simulink model "battery_system_CV_PID"  (R2022a)
settings: Solver=VariableStepAuto  StartTime=0.0  StopTime=10.0  RelTol=1e-3
model workspace (MAT data in the model file):
  AN : object (value not decoded)
  C = [0 0 -0.999999993923 0 0 0 0 0 0 0 0 0 ... (355 elements, 1x355)]
  CA : object (value not decoded)
  CONS : object (value not decoded)
  CV_ref = 3.74905480499
  EL : object (value not decoded)
  FLAG : object (value not decoded)
  K_D = 0
  K_I = -7437.93380511
  K_P = 0
  K_algb = [0 0 0 0 0 0 0 0 0 0 0 0 ... (126025 elements, 355x355)]
  M_cross = [1 0 0 0 0 0 0 0 0 0 0 0 ... (126025 elements, 355x355)]
  N : object (value not decoded)
  P : object (value not decoded)
  PROPS = [100 0.28 0.00733702042142 0.6 2266 720 7.5e-11 1 0.363 3e-13 3e-13 3e-13 ... (475 elements, 19x25)]
  SEP : object (value not decoded)
  SIM : object (value not decoded)
  SV_IC = [298.15 0.0999631520085 0 -0.101224623555 -0.102074642283 -0.171932402214 0.987757586119 14.5346948901 14.535438374 14.5369252829 14.5391554953 14.5421288288 ... (355 elements, 355x1)]
  SampTime = 2
  U_NV_NT = [0 0 0 0 0 0 0 0 0 0 0 0 ... (126025 elements, 355x355)]
  i_user_IC = -1.22418576599
values from neighbouring files (symbols this model uses):
  SIM = rmfield(SIM,'fsolve_options')    [runCC.m]    (also in runCVHold.m = rmfield(SIM,'Controller_MO_File'))
symbols that are objects in the model workspace (value not decoded): AN, CA, CONS, EL, FLAG, N, P, SEP
(part 2 of 2)

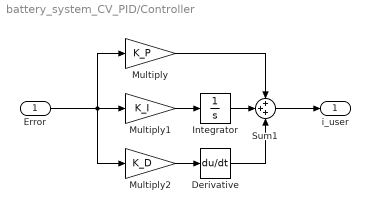
== system battery_system_CV_PID/Controller ==
  Error : Inport
  Derivative : Derivative
  Integrator : Integrator  InitialCondition=i_user_IC
  Multiply : Gain  Gain=K_P
  Multiply1 : Gain  Gain=K_I
  Multiply2 : Gain  Gain=K_D
  Sum1 : Sum  Inputs=+++
  i_user : Outport
  wires:
  Multiply/1 -> Sum1/1
  Integrator/1 -> Sum1/2
  Multiply1/1 -> Integrator/1
  Derivative/1 -> Sum1/3
  Multiply2/1 -> Derivative/1
  Error/1 -> Multiply/1, Multiply2/1, Multiply1/1
  Sum1/1 -> i_user/1

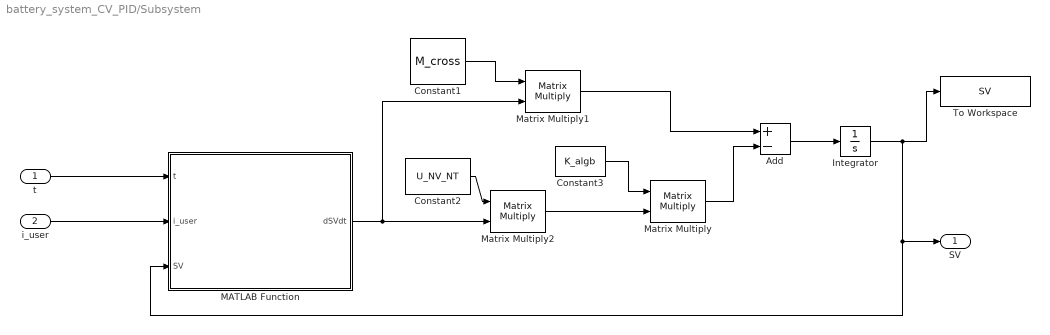
== system battery_system_CV_PID/Subsystem ==
  t : Inport
  i_user : Inport  Port=2
  Add : Sum  Inputs=+-
  Constant1 : Constant  Value=M_cross  VectorParams1D=off
  Constant2 : Constant  Value=U_NV_NT  VectorParams1D=off
  Constant3 : Constant  Value=K_algb  VectorParams1D=off
  Integrator : Integrator  InitialCondition=SV_IC
  MATLAB Function : MATLAB Function  TreatAsAtomicUnit=on
  Matrix Multiply : Product  Multiplication=Matrix(*)
  Matrix Multiply1 : Product  Multiplication=Matrix(*)
  Matrix Multiply2 : Product  Multiplication=Matrix(*)
  To Workspace : ToWorkspace  VariableName=SV  SampleTime=SampTime
  SV : Outport
  wires:
  Add/1 -> Integrator/1
  t/1 -> MATLAB Function/1(t)
  Matrix Multiply/1 -> Add/2
  Constant3/1 -> Matrix Multiply/1
  Constant1/1 -> Matrix Multiply1/1
  Constant2/1 -> Matrix Multiply2/1
  Matrix Multiply1/1 -> Add/1
  MATLAB Function/1(dSVdt) -> Matrix Multiply2/2, Matrix Multiply1/2
  Matrix Multiply2/1 -> Matrix Multiply/2
  Integrator/1 -> SV/1, MATLAB Function/3(SV), To Workspace/1
  i_user/1 -> MATLAB Function/2(i_user)

== matlab function battery_system_CV_PID/Subsystem/MATLAB Function ==
  data: t input; i_user input; dSVdt output; SV input; AN parameter; CA parameter; SEP parameter; EL parameter; SIM parameter; CONS parameter; P parameter; N parameter; FLAG parameter; PROPS parameter
function dSVdt = CallGovnEqns(t,i_user,SV, AN, CA, SEP, EL, SIM, CONS, P, N, FLAG, PROPS)
% Initialize Output
dSVdt = zeros(N.N_SV_tot,1);

% Call GovnEqns
coder.extrinsic('ConvertStrCallGov')
[dSVdt] = ConvertStrCallGov(t,SV,AN,CA,SEP,EL,SIM,CONS,P,N,FLAG,PROPS,i_user);

end
